simulink model "VehicleEx2Part2"  (R2024b)
settings: Solver=VariableStepAuto  StartTime=0.0  StopTime=10.0  RelTol=1e-3
values from neighbouring files (symbols this model uses):
  c1 = 2/10    (= 0.2)    [TireModel_Parameters.m]
  c2 = 6628/1000    (= 6.628)    [TireModel_Parameters.m]
  c3 = 0    [TireModel_Parameters.m]
settings Model: Creator=erona  LastModifiedBy=erona

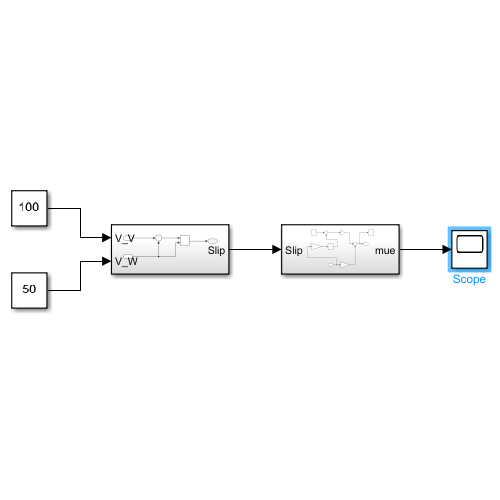
[thumbnail: Simulink's stored preview of the top-level diagram]
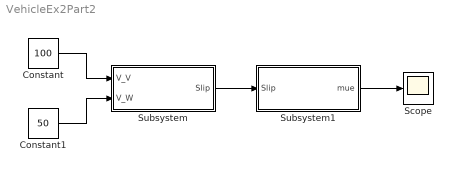
== system VehicleEx2Part2 ==
  Constant : Constant  Value=100
  Constant1 : Constant  Value=50
  Scope : Scope
  Subsystem : Subsystem
  Subsystem1 : Subsystem
  wires:
  Subsystem/1(Slip) -> Subsystem1/1(Slip)
  Constant1/1 -> Subsystem/2(V_W)
  Constant/1 -> Subsystem/1(V_V)
  Subsystem1/1(mue) -> Scope/1

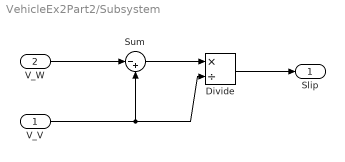
== system VehicleEx2Part2/Subsystem ==
  V_V : Inport
  V_W : Inport  Port=2
  Divide : Product  Inputs=*/
  Sum : Sum  Inputs=|-+
  Slip : Outport
  wires:
  Divide/1 -> Slip/1
  V_W/1 -> Sum/1
  V_V/1 -> Divide/2, Sum/2
  Sum/1 -> Divide/1

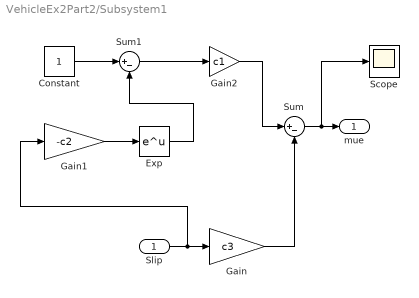
== system VehicleEx2Part2/Subsystem1 ==
  Slip : Inport
  Constant : Constant
  Exp : Math
  Gain : Gain  Gain=c3
  Gain1 : Gain  Gain=-c2
  Gain2 : Gain  Gain=c1
  Scope : Scope
  Sum : Sum  Inputs=|+-
  Sum1 : Sum  Inputs=|+-
  mue : Outport
  wires:
  Slip/1 -> Gain1/1, Gain/1
  Gain/1 -> Sum/2
  Gain1/1 -> Exp/1
  Constant/1 -> Sum1/1
  Exp/1 -> Sum1/2
  Sum1/1 -> Gain2/1
  Gain2/1 -> Sum/1
  Sum/1 -> Scope/1, mue/1
